simulink model "BMS_Advanced_Protection_Algorithm_Design"  (R2024a)
settings: Solver=VariableStepAuto  StartTime=0.0  StopTime=inf  RelTol=1e-3
libraries: simulink x3
settings Model: Creator=gopin  LastModifiedBy=gopin

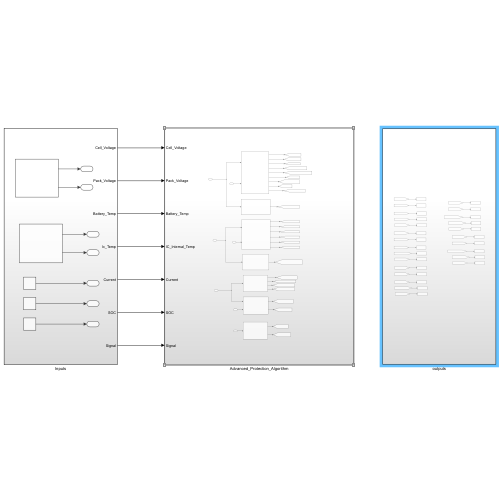
[thumbnail: Simulink's stored preview of the top-level diagram]
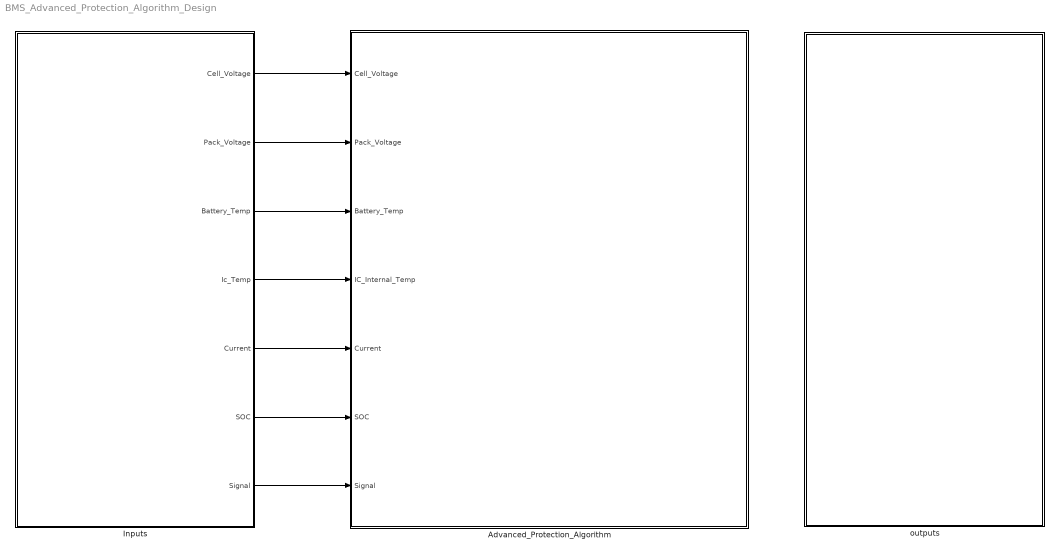
== system BMS_Advanced_Protection_Algorithm_Design ==
  Advanced_Protection_Algorithm : Subsystem
  Inputs : Subsystem
  outputs : Subsystem
  wires:
  Inputs/1(Cell_Voltage) -> Advanced_Protection_Algorithm/1(Cell_Voltage)
  Inputs/2(Pack_Voltage) -> Advanced_Protection_Algorithm/2(Pack_Voltage)
  Inputs/3(Battery_Temp) -> Advanced_Protection_Algorithm/3(Battery_Temp)
  Inputs/4(Ic_Temp) -> Advanced_Protection_Algorithm/4(IC_Internal_Temp)
  Inputs/5(Current) -> Advanced_Protection_Algorithm/5(Current)
  Inputs/6(SOC) -> Advanced_Protection_Algorithm/6(SOC)
  Inputs/7(Signal) -> Advanced_Protection_Algorithm/7(Signal)

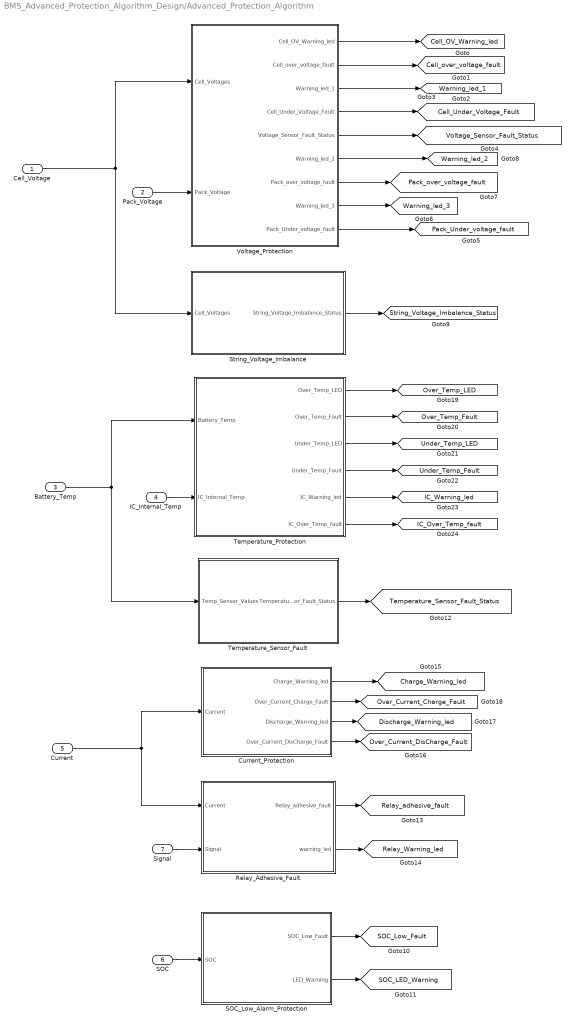
== system BMS_Advanced_Protection_Algorithm_Design/Advanced_Protection_Algorithm ==
  Cell_Voltage : Inport
  Pack_Voltage : Inport  Port=2
  Battery_Temp : Inport  Port=3
  IC_Internal_Temp : Inport  Port=4
  Current : Inport  Port=5
  SOC : Inport  Port=6
  Signal : Inport  Port=7
  Current_Protection : Subsystem
  Relay_Adhesive_Fault : Subsystem
  SOC_Low_Alarm_Protection : Subsystem
  String_Voltage_Imbalance : Subsystem
  Temperature_Protection : Subsystem
  Temperature_Sensor_Fault : Subsystem
  Voltage_Protection : Subsystem
  tag scope: Cell_OV_Warning_led=global, Cell_Under_Voltage_Fault=global, Cell_over_voltage_fault=global, Charge_Warning_led=global, Discharge_Warning_led=global, IC_Over_Temp_fault=global, IC_Warning_led=global, Over_Current_Charge_Fault=global, Over_Current_DisCharge_Fault=global, Over_Temp_Fault=global, Over_Temp_LED=global, Pack_Under_voltage_fault=global, Pack_over_voltage_fault=global, Relay_Warning_led=global, Relay_adhesive_fault=global, SOC_LED_Warning=global, SOC_Low_Fault=global, String_Voltage_Imbalance_Status=global, Temperature_Sensor_Fault_Status=global, Under_Temp_Fault=global, Under_Temp_LED=global, Voltage_Sensor_Fault_Status=global, Warning_led_1=global, Warning_led_2=global, Warning_led_3=global
  wires:
  Current_Protection/4(Over_Current_DisCharge_Fault) -> [Over_Current_DisCharge_Fault]
  Temperature_Protection/4(Under_Temp_Fault) -> [Under_Temp_Fault]
  Signal/1 -> Relay_Adhesive_Fault/2(Signal)
  Current/1 -> Current_Protection/1(Current), Relay_Adhesive_Fault/1(Current)
  Temperature_Sensor_Fault/1(Temperature_Sensor_Fault_Status) -> [Temperature_Sensor_Fault_Status]
  Relay_Adhesive_Fault/1(Relay_adhesive_fault) -> [Relay_adhesive_fault]
  Temperature_Protection/1(Over_Temp_LED) -> [Over_Temp_LED]
  Relay_Adhesive_Fault/2(warning_led) -> [Relay_Warning_led]
  Current_Protection/2(Over_Current_Charge_Fault) -> [Over_Current_Charge_Fault]
  Cell_Voltage/1 -> Voltage_Protection/1(Cell_Voltages), String_Voltage_Imbalance/1(Cell_Voltages)
  Pack_Voltage/1 -> Voltage_Protection/2(Pack_Voltage)
  Temperature_Protection/2(Over_Temp_Fault) -> [Over_Temp_Fault]
  String_Voltage_Imbalance/1(String_Voltage_Imbalance_Status) -> [String_Voltage_Imbalance_Status]
  SOC_Low_Alarm_Protection/1(SOC_Low_Fault) -> [SOC_Low_Fault]
  SOC/1 -> SOC_Low_Alarm_Protection/1(SOC)
  IC_Internal_Temp/1 -> Temperature_Protection/2(IC_Internal_Temp)
  Temperature_Protection/3(Under_Temp_LED) -> [Under_Temp_LED]
  SOC_Low_Alarm_Protection/2(LED_Warning) -> [SOC_LED_Warning]
  Current_Protection/3(Discharge_Warning_led) -> [Discharge_Warning_led]
  Voltage_Protection/1(Cell_OV_Warning_led) -> [Cell_OV_Warning_led]
  Voltage_Protection/3(Warning_led_1) -> [Warning_led_1]
  Voltage_Protection/5(Voltage_Sensor_Fault_Status) -> [Voltage_Sensor_Fault_Status]
  Voltage_Protection/6(Warning_led_2) -> [Warning_led_2]
  Voltage_Protection/7(Pack_over_voltage_fault) -> [Pack_over_voltage_fault]
  Voltage_Protection/8(Warning_led_3) -> [Warning_led_3]
  Temperature_Protection/5(IC_Warning_led) -> [IC_Warning_led]
  Temperature_Protection/6(IC_Over_Temp_fault) -> [IC_Over_Temp_fault]
  Battery_Temp/1 -> Temperature_Protection/1(Battery_Temp), Temperature_Sensor_Fault/1(Temp_Sensor_Values)
  Voltage_Protection/2(Cell_over_voltage_fault) -> [Cell_over_voltage_fault]
  Voltage_Protection/4(Cell_Under_Voltage_Fault) -> [Cell_Under_Voltage_Fault]
  Voltage_Protection/9(Pack_Under_voltage_fault) -> [Pack_Under_voltage_fault]
  Current_Protection/1(Charge_Warning_led) -> [Charge_Warning_led]

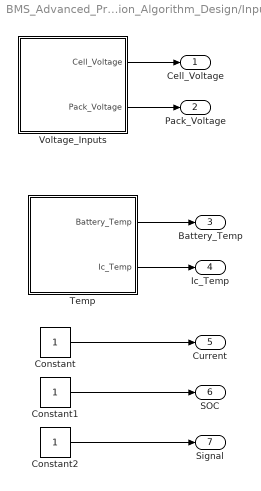
== system BMS_Advanced_Protection_Algorithm_Design/Inputs ==
  Constant : Constant
  Constant1 : Constant
  Constant2 : Constant
  Temp : Subsystem
  Voltage_Inputs : Subsystem
  Cell_Voltage : Outport
  Pack_Voltage : Outport  Port=2
  Battery_Temp : Outport  Port=3
  Ic_Temp : Outport  Port=4
  Current : Outport  Port=5
  SOC : Outport  Port=6
  Signal : Outport  Port=7
  wires:
  Voltage_Inputs/1(Cell_Voltage) -> Cell_Voltage/1
  Voltage_Inputs/2(Pack_Voltage) -> Pack_Voltage/1
  Temp/1(Battery_Temp) -> Battery_Temp/1
  Temp/2(Ic_Temp) -> Ic_Temp/1
  Constant/1 -> Current/1
  Constant1/1 -> SOC/1
  Constant2/1 -> Signal/1

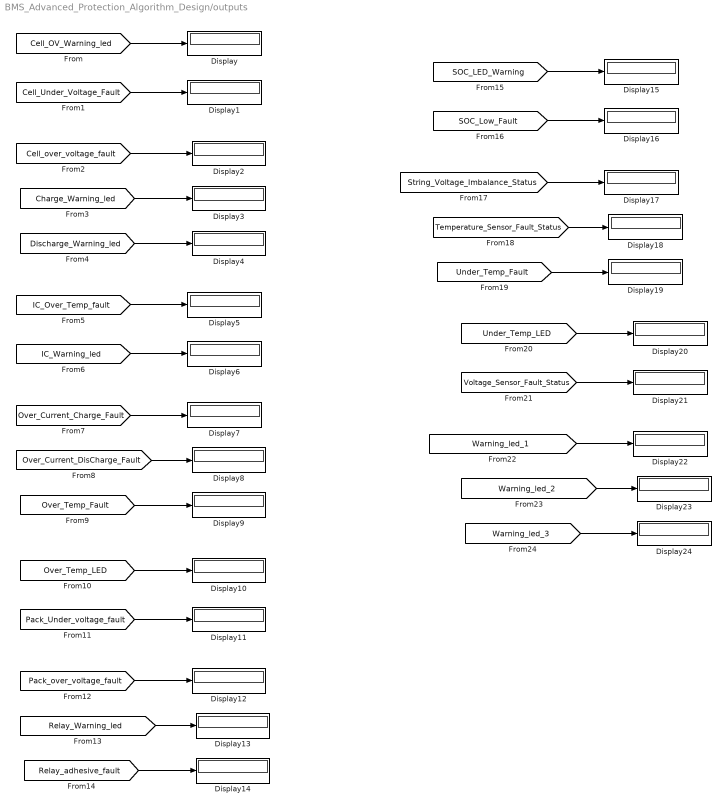
== system BMS_Advanced_Protection_Algorithm_Design/outputs ==
  Display{,1..24} (25 alike) : Display
  wires:
  [Cell_OV_Warning_led] -> Display/1
  [Cell_Under_Voltage_Fault] -> Display1/1
  [Cell_over_voltage_fault] -> Display2/1
  [Charge_Warning_led] -> Display3/1
  [Discharge_Warning_led] -> Display4/1
  [IC_Warning_led] -> Display6/1
  [Over_Current_Charge_Fault] -> Display7/1
  [Over_Current_DisCharge_Fault] -> Display8/1
  [Over_Temp_Fault] -> Display9/1
  [IC_Over_Temp_fault] -> Display5/1
  [Relay_adhesive_fault] -> Display14/1
  [Relay_Warning_led] -> Display13/1
  [Pack_over_voltage_fault] -> Display12/1
  [Over_Temp_LED] -> Display10/1
  [Pack_Under_voltage_fault] -> Display11/1
  [SOC_LED_Warning] -> Display15/1
  [String_Voltage_Imbalance_Status] -> Display17/1
  [Under_Temp_Fault] -> Display19/1
  [SOC_Low_Fault] -> Display16/1
  [Temperature_Sensor_Fault_Status] -> Display18/1
  [Warning_led_2] -> Display23/1
  [Warning_led_1] -> Display22/1
  [Voltage_Sensor_Fault_Status] -> Display21/1
  [Warning_led_3] -> Display24/1
  [Under_Temp_LED] -> Display20/1

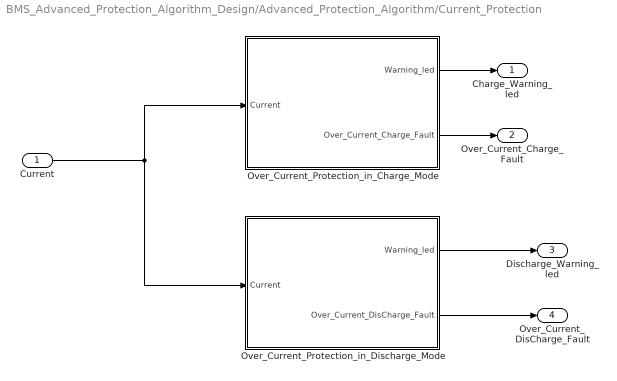
== system BMS_Advanced_Protection_Algorithm_Design/Advanced_Protection_Algorithm/Current_Protection ==
  Current : Inport
  Over_Current_Protection_in_Charge_Mode : Subsystem
  Over_Current_Protection_in_Discharge_Mode : Subsystem
  Charge_Warning_led : Outport
  Over_Current_Charge_Fault : Outport  Port=2
  Discharge_Warning_led : Outport  Port=3
  Over_Current_DisCharge_Fault : Outport  Port=4
  wires:
  Over_Current_Protection_in_Charge_Mode/1(Warning_led) -> Charge_Warning_led/1
  Over_Current_Protection_in_Charge_Mode/2(Over_Current_Charge_Fault) -> Over_Current_Charge_Fault/1
  Over_Current_Protection_in_Discharge_Mode/2(Over_Current_DisCharge_Fault) -> Over_Current_DisCharge_Fault/1
  Over_Current_Protection_in_Discharge_Mode/1(Warning_led) -> Discharge_Warning_led/1
  Current/1 -> Over_Current_Protection_in_Discharge_Mode/1(Current), Over_Current_Protection_in_Charge_Mode/1(Current)

== system BMS_Advanced_Protection_Algorithm_Design/Advanced_Protection_Algorithm/Relay_Adhesive_Fault ==
  Current : Inport
  Signal : Inport  Port=2
  Chart : Stateflow chart  TreatAsAtomicUnit=on
  Relay_adhesive_fault : Outport
  warning_led : Outport  Port=2
  wires:
  Current/1 -> Chart/1(Current)
  Signal/1 -> Chart/2(Signal)
  Chart/1(relay_adhesive_fault) -> Relay_adhesive_fault/1
  Chart/2(warning_led) -> warning_led/1

== system BMS_Advanced_Protection_Algorithm_Design/Advanced_Protection_Algorithm/SOC_Low_Alarm_Protection ==
  SOC : Inport
  Chart : Stateflow chart  TreatAsAtomicUnit=on
  SOC_Low_Fault : Outport
  LED_Warning : Outport  Port=2
  wires:
  Chart/1(SOC_Low_Fault) -> SOC_Low_Fault/1
  SOC/1 -> Chart/1(SOC)
  Chart/2(warning_led) -> LED_Warning/1

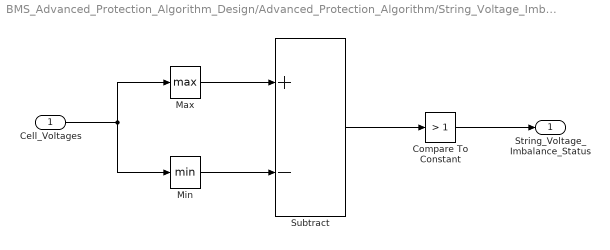
== system BMS_Advanced_Protection_Algorithm_Design/Advanced_Protection_Algorithm/String_Voltage_Imbalance ==
  Cell_Voltages : Inport
  Compare To Constant : simulink/Logic and Bit Operations/Compare To Constant  relop=>  const=1  OutDataTypeStr=boolean
  Max : MinMax  Function=max
  Min : MinMax
  Subtract : Sum  Inputs=+-
  String_Voltage_Imbalance_Status : Outport
  wires:
  Subtract/1 -> Compare To Constant/1
  Compare To Constant/1 -> String_Voltage_Imbalance_Status/1
  Min/1 -> Subtract/2
  Max/1 -> Subtract/1
  Cell_Voltages/1 -> Min/1, Max/1

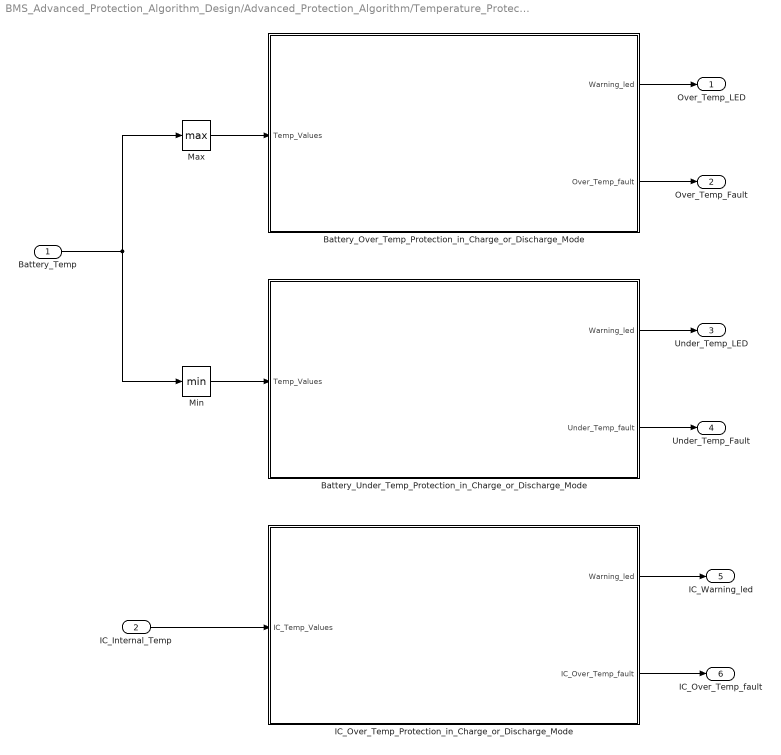
== system BMS_Advanced_Protection_Algorithm_Design/Advanced_Protection_Algorithm/Temperature_Protection ==
  Battery_Temp : Inport
  IC_Internal_Temp : Inport  Port=2
  Battery_Over_Temp_Protection_in_Charge_or_Discharge_Mode : Subsystem
  Battery_Under_Temp_Protection_in_Charge_or_Discharge_Mode : Subsystem
  IC_Over_Temp_Protection_in_Charge_or_Discharge_Mode : Subsystem
  Max : MinMax  Function=max
  Min : MinMax
  Over_Temp_LED : Outport
  Over_Temp_Fault : Outport  Port=2
  Under_Temp_LED : Outport  Port=3
  Under_Temp_Fault : Outport  Port=4
  IC_Warning_led : Outport  Port=5
  IC_Over_Temp_fault : Outport  Port=6
  wires:
  Battery_Over_Temp_Protection_in_Charge_or_Discharge_Mode/1(Warning_led) -> Over_Temp_LED/1
  Battery_Over_Temp_Protection_in_Charge_or_Discharge_Mode/2(Over_Temp_fault) -> Over_Temp_Fault/1
  Max/1 -> Battery_Over_Temp_Protection_in_Charge_or_Discharge_Mode/1(Temp_Values)
  Min/1 -> Battery_Under_Temp_Protection_in_Charge_or_Discharge_Mode/1(Temp_Values)
  Battery_Temp/1 -> Min/1, Max/1
  Battery_Under_Temp_Protection_in_Charge_or_Discharge_Mode/1(Warning_led) -> Under_Temp_LED/1
  Battery_Under_Temp_Protection_in_Charge_or_Discharge_Mode/2(Under_Temp_fault) -> Under_Temp_Fault/1
  IC_Internal_Temp/1 -> IC_Over_Temp_Protection_in_Charge_or_Discharge_Mode/1(IC_Temp_Values)
  IC_Over_Temp_Protection_in_Charge_or_Discharge_Mode/1(Warning_led) -> IC_Warning_led/1
  IC_Over_Temp_Protection_in_Charge_or_Discharge_Mode/2(IC_Over_Temp_fault) -> IC_Over_Temp_fault/1

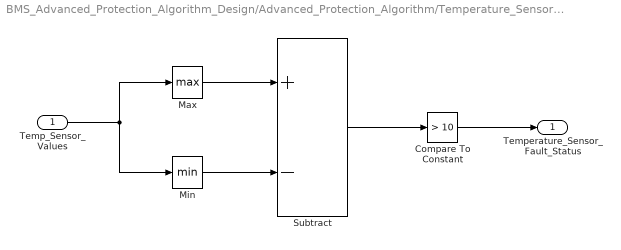
== system BMS_Advanced_Protection_Algorithm_Design/Advanced_Protection_Algorithm/Temperature_Sensor_Fault ==
  Temp_Sensor_Values : Inport
  Compare To Constant : simulink/Logic and Bit Operations/Compare To Constant  relop=>  const=10  OutDataTypeStr=boolean
  Max : MinMax  Function=max
  Min : MinMax
  Subtract : Sum  Inputs=+-
  Temperature_Sensor_Fault_Status : Outport
  wires:
  Temp_Sensor_Values/1 -> Min/1, Max/1
  Max/1 -> Subtract/1
  Min/1 -> Subtract/2
  Subtract/1 -> Compare To Constant/1
  Compare To Constant/1 -> Temperature_Sensor_Fault_Status/1

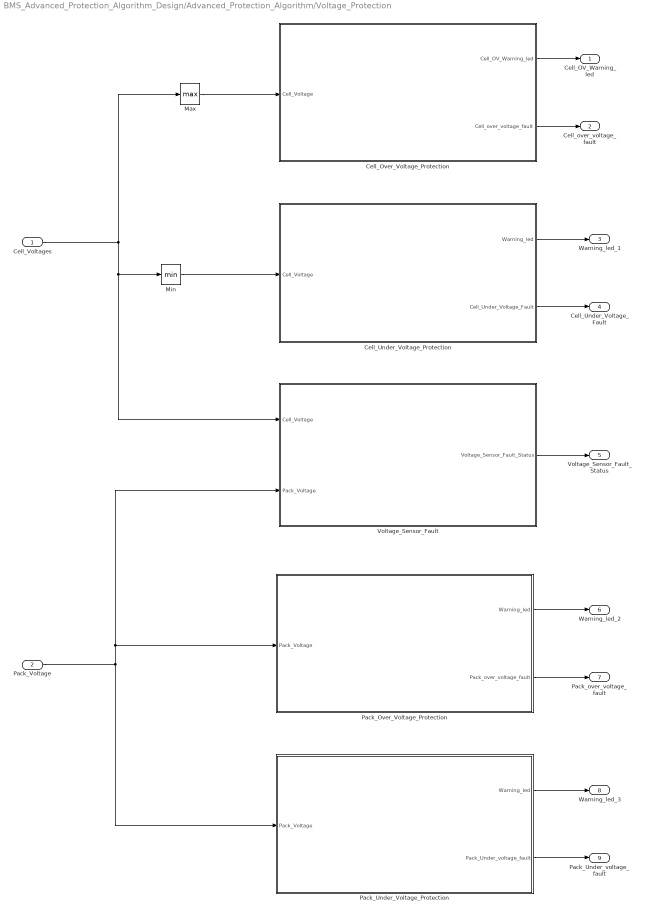
== system BMS_Advanced_Protection_Algorithm_Design/Advanced_Protection_Algorithm/Voltage_Protection ==
  Cell_Voltages : Inport
  Pack_Voltage : Inport  Port=2
  Cell_Over_Voltage_Protection : Subsystem
  Cell_Under_Voltage_Protection : Subsystem
  Max : MinMax  Function=max
  Min : MinMax
  Pack_Over_Voltage_Protection : Subsystem
  Pack_Under_Voltage_Protection : Subsystem
  Voltage_Sensor_Fault : Subsystem
  Cell_OV_Warning_led : Outport
  Cell_over_voltage_fault : Outport  Port=2
  Warning_led_1 : Outport  Port=3
  Cell_Under_Voltage_Fault : Outport  Port=4
  Voltage_Sensor_Fault_Status : Outport  Port=5
  Warning_led_2 : Outport  Port=6
  Pack_over_voltage_fault : Outport  Port=7
  Warning_led_3 : Outport  Port=8
  Pack_Under_voltage_fault : Outport  Port=9
  wires:
  Max/1 -> Cell_Over_Voltage_Protection/1(Cell_Voltage)
  Min/1 -> Cell_Under_Voltage_Protection/1(Cell_Voltage)
  Cell_Voltages/1 -> Max/1, Voltage_Sensor_Fault/1(Cell_Voltage), Min/1
  Pack_Voltage/1 -> Pack_Under_Voltage_Protection/1(Pack_Voltage), Pack_Over_Voltage_Protection/1(Pack_Voltage), Voltage_Sensor_Fault/2(Pack_Voltage)
  Cell_Over_Voltage_Protection/1(Cell_OV_Warning_led) -> Cell_OV_Warning_led/1
  Cell_Over_Voltage_Protection/2(Cell_over_voltage_fault) -> Cell_over_voltage_fault/1
  Cell_Under_Voltage_Protection/1(Warning_led) -> Warning_led_1/1
  Cell_Under_Voltage_Protection/2(Cell_Under_Voltage_Fault) -> Cell_Under_Voltage_Fault/1
  Voltage_Sensor_Fault/1(Voltage_Sensor_Fault_Status) -> Voltage_Sensor_Fault_Status/1
  Pack_Over_Voltage_Protection/1(Warning_led) -> Warning_led_2/1
  Pack_Over_Voltage_Protection/2(Pack_over_voltage_fault) -> Pack_over_voltage_fault/1
  Pack_Under_Voltage_Protection/1(Warning_led) -> Warning_led_3/1
  Pack_Under_Voltage_Protection/2(Pack_Under_voltage_fault) -> Pack_Under_voltage_fault/1

== system BMS_Advanced_Protection_Algorithm_Design/Inputs/Temp ==
  Battery_Temperature : Subsystem
  Constant : Constant
  Mux : Mux  Inputs=7
  Battery_Temp : Outport
  Ic_Temp : Outport  Port=2
  wires:
  Mux/1 -> Battery_Temp/1
  Battery_Temperature/1(Outport) -> Mux/1
  Battery_Temperature/2(Outport1) -> Mux/2
  Battery_Temperature/3(Outport2) -> Mux/3
  Battery_Temperature/4(Outport3) -> Mux/4
  Battery_Temperature/5(Outport4) -> Mux/5
  Battery_Temperature/6(Outport5) -> Mux/6
  Battery_Temperature/7(Outport6) -> Mux/7
  Constant/1 -> Ic_Temp/1

== system BMS_Advanced_Protection_Algorithm_Design/Inputs/Voltage_Inputs ==
  Cell_Voltages : Subsystem
  Constant : Constant
  Mux : Mux  Inputs=14
  Cell_Voltage : Outport
  Pack_Voltage : Outport  Port=2
  wires:
  Constant/1 -> Pack_Voltage/1
  Mux/1 -> Cell_Voltage/1
  Cell_Voltages/1(Outport) -> Mux/1
  Cell_Voltages/2(Outport1) -> Mux/2
  Cell_Voltages/3(Outport2) -> Mux/3
  Cell_Voltages/4(Outport3) -> Mux/4
  Cell_Voltages/5(Outport4) -> Mux/5
  Cell_Voltages/6(Outport5) -> Mux/6
  Cell_Voltages/7(Outport6) -> Mux/7
  Cell_Voltages/8(Outport7) -> Mux/8
  Cell_Voltages/9(Outport8) -> Mux/9
  Cell_Voltages/10(Outport9) -> Mux/10
  Cell_Voltages/11(Outport10) -> Mux/11
  Cell_Voltages/12(Outport11) -> Mux/12
  Cell_Voltages/13(Outport12) -> Mux/13
  Cell_Voltages/14(Outport13) -> Mux/14

== system BMS_Advanced_Protection_Algorithm_Design/Advanced_Protection_Algorithm/Current_Protection/Over_Current_Protection_in_Charge_Mode ==
  Current : Inport
  Over_Current_Protection_in_Charge_Mode : Stateflow chart  TreatAsAtomicUnit=on
  Warning_led : Outport
  Over_Current_Charge_Fault : Outport  Port=2
  wires:
  Current/1 -> Over_Current_Protection_in_Charge_Mode/1(Current)
  Over_Current_Protection_in_Charge_Mode/1(Warning_led) -> Warning_led/1
  Over_Current_Protection_in_Charge_Mode/2(Over_Current_Charge_Fault) -> Over_Current_Charge_Fault/1

== system BMS_Advanced_Protection_Algorithm_Design/Advanced_Protection_Algorithm/Current_Protection/Over_Current_Protection_in_Discharge_Mode ==
  Current : Inport
  Over_Current_Protection_in_DisCharge_Mode : Stateflow chart  TreatAsAtomicUnit=on
  Warning_led : Outport
  Over_Current_DisCharge_Fault : Outport  Port=2
  wires:
  Current/1 -> Over_Current_Protection_in_DisCharge_Mode/1(Current)
  Over_Current_Protection_in_DisCharge_Mode/1(Warning_led) -> Warning_led/1
  Over_Current_Protection_in_DisCharge_Mode/2(Over_Current_DisCharge_Fault) -> Over_Current_DisCharge_Fault/1

== system BMS_Advanced_Protection_Algorithm_Design/Advanced_Protection_Algorithm/Temperature_Protection/Battery_Over_Temp_Protection_in_Charge_or_Discharge_Mode ==
  Temp_Values : Inport
  Over_Temp_Protection : Stateflow chart  TreatAsAtomicUnit=on
  Warning_led : Outport
  Over_Temp_fault : Outport  Port=2
  wires:
  Over_Temp_Protection/1(Warning_led) -> Warning_led/1
  Temp_Values/1 -> Over_Temp_Protection/1(Max_Temp_data)
  Over_Temp_Protection/2(Over_Temp_fault) -> Over_Temp_fault/1

== system BMS_Advanced_Protection_Algorithm_Design/Advanced_Protection_Algorithm/Temperature_Protection/Battery_Under_Temp_Protection_in_Charge_or_Discharge_Mode ==
  Temp_Values : Inport
  Under_Temp_Protection : Stateflow chart  TreatAsAtomicUnit=on
  Warning_led : Outport
  Under_Temp_fault : Outport  Port=2
  wires:
  Under_Temp_Protection/1(Warning_led) -> Warning_led/1
  Temp_Values/1 -> Under_Temp_Protection/1(Min_Temp_data)
  Under_Temp_Protection/2(Under_Temp_fault) -> Under_Temp_fault/1

== system BMS_Advanced_Protection_Algorithm_Design/Advanced_Protection_Algorithm/Temperature_Protection/IC_Over_Temp_Protection_in_Charge_or_Discharge_Mode ==
  IC_Temp_Values : Inport
  IC_Over_Temp_Protection : Stateflow chart  TreatAsAtomicUnit=on
  Warning_led : Outport
  IC_Over_Temp_fault : Outport  Port=2
  wires:
  IC_Over_Temp_Protection/1(Warning_led) -> Warning_led/1
  IC_Over_Temp_Protection/2(IC_Over_Temp_fault) -> IC_Over_Temp_fault/1
  IC_Temp_Values/1 -> IC_Over_Temp_Protection/1(IC_Temp_data)

== system BMS_Advanced_Protection_Algorithm_Design/Advanced_Protection_Algorithm/Voltage_Protection/Cell_Over_Voltage_Protection ==
  Cell_Voltage : Inport
  Over_Voltage_Protection : Stateflow chart  TreatAsAtomicUnit=on
  Cell_OV_Warning_led : Outport
  Cell_over_voltage_fault : Outport  Port=2
  wires:
  Cell_Voltage/1 -> Over_Voltage_Protection/1(Cell_Voltage)
  Over_Voltage_Protection/2(Cell_over_voltage_fault) -> Cell_over_voltage_fault/1
  Over_Voltage_Protection/1(Warning_led) -> Cell_OV_Warning_led/1

== system BMS_Advanced_Protection_Algorithm_Design/Advanced_Protection_Algorithm/Voltage_Protection/Cell_Under_Voltage_Protection ==
  Cell_Voltage : Inport
  Under_Voltage_Protection : Stateflow chart  TreatAsAtomicUnit=on
  Warning_led : Outport
  Cell_Under_Voltage_Fault : Outport  Port=2
  wires:
  Cell_Voltage/1 -> Under_Voltage_Protection/1(Cell_Voltage)
  Under_Voltage_Protection/1(Warning_led) -> Warning_led/1
  Under_Voltage_Protection/2(Cell_Under_voltage_fault) -> Cell_Under_Voltage_Fault/1

== system BMS_Advanced_Protection_Algorithm_Design/Advanced_Protection_Algorithm/Voltage_Protection/Pack_Over_Voltage_Protection ==
  Pack_Voltage : Inport
  Over_Voltage_Protection : Stateflow chart  TreatAsAtomicUnit=on
  Warning_led : Outport
  Pack_over_voltage_fault : Outport  Port=2
  wires:
  Over_Voltage_Protection/1(Warning_led) -> Warning_led/1
  Pack_Voltage/1 -> Over_Voltage_Protection/1(Pack_Voltage)
  Over_Voltage_Protection/2(Pack_over_voltage_fault) -> Pack_over_voltage_fault/1

== system BMS_Advanced_Protection_Algorithm_Design/Advanced_Protection_Algorithm/Voltage_Protection/Pack_Under_Voltage_Protection ==
  Pack_Voltage : Inport
  Under_Voltage_Protection : Stateflow chart  TreatAsAtomicUnit=on
  Warning_led : Outport
  Pack_Under_voltage_fault : Outport  Port=2
  wires:
  Under_Voltage_Protection/1(Warning_led) -> Warning_led/1
  Pack_Voltage/1 -> Under_Voltage_Protection/1(Pack_Voltage)
  Under_Voltage_Protection/2(Pack_Under_voltage_fault) -> Pack_Under_voltage_fault/1

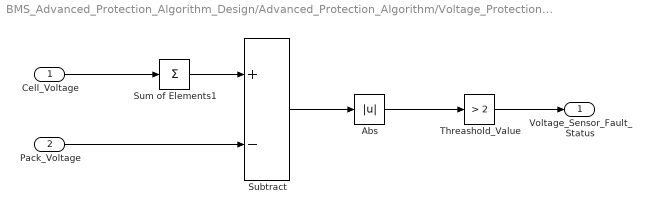
== system BMS_Advanced_Protection_Algorithm_Design/Advanced_Protection_Algorithm/Voltage_Protection/Voltage_Sensor_Fault ==
  Cell_Voltage : Inport
  Pack_Voltage : Inport  Port=2
  Abs : Abs  SaturateOnIntegerOverflow=off
  Subtract : Sum  Inputs=+-
  Sum of Elements1 : Sum  Inputs=+
  Threashold_Value : simulink/Logic and Bit Operations/Compare To Constant  relop=>  const=2  OutDataTypeStr=boolean
  Voltage_Sensor_Fault_Status : Outport
  wires:
  Cell_Voltage/1 -> Sum of Elements1/1
  Pack_Voltage/1 -> Subtract/2
  Sum of Elements1/1 -> Subtract/1
  Subtract/1 -> Abs/1
  Abs/1 -> Threashold_Value/1
  Threashold_Value/1 -> Voltage_Sensor_Fault_Status/1

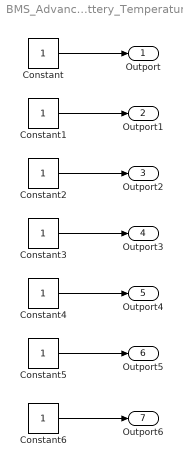
== system BMS_Advanced_Protection_Algorithm_Design/Inputs/Temp/Battery_Temperature ==
  Constant{,1..6} (7 alike) : Constant
  Outport : Outport
  Outport1 : Outport  Port=2
  Outport2 : Outport  Port=3
  Outport3 : Outport  Port=4
  Outport4 : Outport  Port=5
  Outport5 : Outport  Port=6
  Outport6 : Outport  Port=7
  wires:
  Constant/1 -> Outport/1
  Constant1/1 -> Outport1/1
  Constant2/1 -> Outport2/1
  Constant3/1 -> Outport3/1
  Constant4/1 -> Outport4/1
  Constant5/1 -> Outport5/1
  Constant6/1 -> Outport6/1

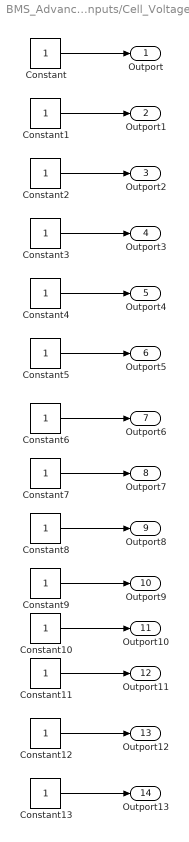
== system BMS_Advanced_Protection_Algorithm_Design/Inputs/Voltage_Inputs/Cell_Voltages ==
  Constant{,1..13} (14 alike) : Constant
  Outport : Outport
  Outport1 : Outport  Port=2
  Outport2 : Outport  Port=3
  Outport3 : Outport  Port=4
  Outport4 : Outport  Port=5
  Outport5 : Outport  Port=6
  Outport6 : Outport  Port=7
  Outport7 : Outport  Port=8
  Outport8 : Outport  Port=9
  Outport9 : Outport  Port=10
  Outport10 : Outport  Port=11
  Outport11 : Outport  Port=12
  Outport12 : Outport  Port=13
  Outport13 : Outport  Port=14
  wires:
  Constant/1 -> Outport/1
  Constant1/1 -> Outport1/1
  Constant2/1 -> Outport2/1
  Constant3/1 -> Outport3/1
  Constant4/1 -> Outport4/1
  Constant5/1 -> Outport5/1
  Constant6/1 -> Outport6/1
  Constant7/1 -> Outport7/1
  Constant8/1 -> Outport8/1
  Constant9/1 -> Outport9/1
  Constant10/1 -> Outport10/1
  Constant11/1 -> Outport11/1
  Constant12/1 -> Outport12/1
  Constant13/1 -> Outport13/1

== stateflow chart BMS_Advanced_Protection_Algorithm_Design/Advanced_Protection_Algorithm/Temperature_Protection/Battery_Over_Temp_Protection_in_Charge_or_Discharge_Mode/Over_Temp_Protection ==
  state Initial_Condition
    en:
    Over_Temp_fault=0;
    Warning_led=0;
  state Level_1_Trigger
    en:
    Over_Temp_fault=1;
    state LED_off
      en:
      Warning_led=0;
    state LED_on
      en:
      Warning_led=1;
    (default) -> LED_off
    LED_off -> LED_on : [after(1,sec)]
    LED_on -> LED_off : [after(1,sec)]
  state Level_3_Trigger
    en:
    Over_Temp_fault=1;
    Warning_led=1;
    du:
    Warning_led=1;
  (default) -> Initial_Condition
  Initial_Condition -> Level_1_Trigger : [Max_Temp_data > 55 && after(5,sec)]
  Level_1_Trigger -> Initial_Condition [order 1] : [Max_Temp_data < 50]
  Level_3_Trigger -> Initial_Condition [order 2] : [Max_Temp_data<50]
  Level_1_Trigger -> Level_3_Trigger [order 2] : [Max_Temp_data>60 && after(3,sec)]
  Level_3_Trigger -> Level_1_Trigger [order 1] : [Max_Temp_data<60]
  data: Warning_led output; Max_Temp_data input; Over_Temp_fault output

== stateflow chart BMS_Advanced_Protection_Algorithm_Design/Advanced_Protection_Algorithm/Temperature_Protection/Battery_Under_Temp_Protection_in_Charge_or_Discharge_Mode/Under_Temp_Protection ==
  state Initial_Condition
    en:
    Under_Temp_fault=0;
    Warning_led=0;
  state Level_1_Trigger
    en:
    Under_Temp_fault=1;
    state LED_off
      en:
      Warning_led=0;
    state LED_on
      en:
      Warning_led=1;
    (default) -> LED_off
    LED_off -> LED_on : [after(1,sec)]
    LED_on -> LED_off : [after(1,sec)]
  state Level_3_Trigger
    en:
    Under_Temp_fault=1;
    Warning_led=1;
    du:
    Warning_led=1;
  (default) -> Initial_Condition
  Initial_Condition -> Level_1_Trigger : [Min_Temp_data < 15 && after(5,sec)]
  Level_1_Trigger -> Initial_Condition [order 1] : [Min_Temp_data > 20]
  Level_3_Trigger -> Initial_Condition [order 2] : [Min_Temp_data>20]
  Level_1_Trigger -> Level_3_Trigger [order 2] : [Min_Temp_data <10 && after(3,sec)]
  Level_3_Trigger -> Level_1_Trigger [order 1] : [Min_Temp_data> 10]
  data: Warning_led output; Min_Temp_data input; Under_Temp_fault output

== stateflow chart BMS_Advanced_Protection_Algorithm_Design/Advanced_Protection_Algorithm/Temperature_Protection/IC_Over_Temp_Protection_in_Charge_or_Discharge_Mode/IC_Over_Temp_Protection ==
  state Initial_Condition
    en:
    IC_Over_Temp_fault=0;
    Warning_led=0;
  state Level_1_Trigger
    en:
    IC_Over_Temp_fault=1;
    state LED_off
      en:
      Warning_led=0;
    state LED_on
      en:
      Warning_led=1;
    (default) -> LED_off
    LED_off -> LED_on : [after(1,sec)]
    LED_on -> LED_off : [after(1,sec)]
  state Level_3_Trigger
    en:
    IC_Over_Temp_fault=1;
    Warning_led=1;
    du:
    Warning_led=1;
  (default) -> Initial_Condition
  Initial_Condition -> Level_1_Trigger : [IC_Temp_data > 60 && after(5,sec)]
  Level_1_Trigger -> Initial_Condition [order 1] : [IC_Temp_data < 55]
  Level_3_Trigger -> Initial_Condition [order 2] : [IC_Temp_data<55]
  Level_1_Trigger -> Level_3_Trigger [order 2] : [IC_Temp_data>70 && after(3,sec)]
  Level_3_Trigger -> Level_1_Trigger [order 1] : [IC_Temp_data<70]
  data: Warning_led output; IC_Over_Temp_fault output; IC_Temp_data input

== stateflow chart BMS_Advanced_Protection_Algorithm_Design/Advanced_Protection_Algorithm/SOC_Low_Alarm_Protection/Chart ==
  state Initial_Condition
    en:
    SOC_Low_Fault=0;
  state Level_1_Warning
    en:
    SOC_Low_Fault=1;
    state LED_off
      en:
      warning_led=0;
    state LED_on
      en:
      warning_led=1;
    (default) -> LED_off
    LED_on -> LED_off : [after(1,sec)]
    LED_off -> LED_on : [after(1,sec)]
  (default) -> Initial_Condition
  Initial_Condition -> Level_1_Warning : [SOC < 10 && after(5,sec)]
  Level_1_Warning -> Initial_Condition : [SOC >10]
  data: SOC_Low_Fault output; warning_led output; SOC input

== stateflow chart BMS_Advanced_Protection_Algorithm_Design/Advanced_Protection_Algorithm/Current_Protection/Over_Current_Protection_in_Charge_Mode/Over_Current_Protection_in_Charge_Mode ==
  state Initial_Condition
    en:
    Over_Current_Charge_Fault=0;
    Warning_led=0;
  state Level_1_Trigger
    en:
    Over_Current_Charge_Fault=1;
    state LED_off
      en:
      Warning_led=0;
    state LED_on
      en:
      Warning_led=1;
    (default) -> LED_off
    LED_off -> LED_on : [after(1,sec)]
    LED_on -> LED_off : [after(1,sec)]
  state Level_3_Trigger
    en:
    Over_Current_Charge_Fault=1;
    Warning_led=1;
    du:
    Warning_led=1;
  (default) -> Initial_Condition
  Initial_Condition -> Level_1_Trigger : [Current > 3 && after(5,sec)]
  Level_1_Trigger -> Initial_Condition [order 1] : [Current < 3]
  Level_3_Trigger -> Initial_Condition [order 2] : [Current < 3]
  Level_1_Trigger -> Level_3_Trigger [order 2] : [Current >4 && after(3,sec)]
  Level_3_Trigger -> Level_1_Trigger [order 1] : [Current <4]
  data: Warning_led output; Over_Current_Charge_Fault output; Current input

== stateflow chart BMS_Advanced_Protection_Algorithm_Design/Advanced_Protection_Algorithm/Current_Protection/Over_Current_Protection_in_Discharge_Mode/Over_Current_Protection_in_DisCharge_Mode ==
  state Initial_Condition
    en:
    Over_Current_DisCharge_Fault=0;
    Warning_led=0;
  state Level_1_Trigger
    en:
    Over_Current_DisCharge_Fault=1;
    state LED_off
      en:
      Warning_led=0;
    state LED_on
      en:
      Warning_led=1;
    (default) -> LED_off
    LED_off -> LED_on : [after(1,sec)]
    LED_on -> LED_off : [after(1,sec)]
  state Level_3_Trigger
    en:
    Over_Current_DisCharge_Fault=1;
    Warning_led=1;
    du:
    Warning_led=1;
  (default) -> Initial_Condition
  Initial_Condition -> Level_1_Trigger : [Current < -5 && after(5,sec)]
  Level_1_Trigger -> Initial_Condition [order 1] : [Current >-5]
  Level_3_Trigger -> Initial_Condition [order 2] : [Current >-5]
  Level_1_Trigger -> Level_3_Trigger [order 2] : [Current < -6 && after(3,sec)]
  Level_3_Trigger -> Level_1_Trigger [order 1] : [Current > -6]
  data: Warning_led output; Current input; Over_Current_DisCharge_Fault output

== stateflow chart BMS_Advanced_Protection_Algorithm_Design/Advanced_Protection_Algorithm/Relay_Adhesive_Fault/Chart ==
  state Cond_1
    en:
    relay_adhesive_fault=0;
  state Cond_2
    en:
    relay_adhesive_fault=1;
    state Led_off
      en:
      warning_led=0;
    state Led_on
      en:
      warning_led=1;
    (default) -> Led_off
    Led_on -> Led_off : [after(1,sec)]
    Led_off -> Led_on : [after(1,sec)]
  (default) -> Cond_1
  Cond_1 -> Cond_2 : [Signal==0 && Current >1]
  Cond_2 -> Cond_1 : [Signal == 0 && Current <1 ]
  data: Current input; Signal input; relay_adhesive_fault output; warning_led output

== stateflow chart BMS_Advanced_Protection_Algorithm_Design/Advanced_Protection_Algorithm/Voltage_Protection/Cell_Under_Voltage_Protection/Under_Voltage_Protection ==
  state Initial_Condition
    en:
    Cell_Under_voltage_fault=0;
    Warning_led=0;
  state Level_1_Trigger
    en:
    Cell_Under_voltage_fault=1;
    state LED_off
      en:
      Warning_led=0;
    state LED_on
      en:
      Warning_led=1;
    (default) -> LED_off
    LED_off -> LED_on : [after(1,sec)]
    LED_on -> LED_off : [after(1,sec)]
  state Level_3_Trigger
    en:
    Cell_Under_voltage_fault=1;
    Warning_led=1;
    du:
    Warning_led=1;
  (default) -> Initial_Condition
  Initial_Condition -> Level_1_Trigger : [Cell_Voltage <3  && after(5,sec)]
  Level_1_Trigger -> Initial_Condition [order 1] : [Cell_Voltage > 3.05]
  Level_3_Trigger -> Initial_Condition [order 2] : [Cell_Voltage > 3.05]
  Level_1_Trigger -> Level_3_Trigger [order 2] : [Cell_Voltage < 2.8 && after(3,sec)]
  Level_3_Trigger -> Level_1_Trigger [order 1] : [Cell_Voltage > 2.85]
  data: Cell_Voltage input; Warning_led output; Cell_Under_voltage_fault output

== stateflow chart BMS_Advanced_Protection_Algorithm_Design/Advanced_Protection_Algorithm/Voltage_Protection/Pack_Over_Voltage_Protection/Over_Voltage_Protection ==
  state Initial_Condition
    en:
    Pack_over_voltage_fault=0;
    Warning_led=0;
  state Level_1_Trigger
    en:
    Pack_over_voltage_fault=1;
    state LED_off
      en:
      Warning_led=0;
    state LED_on
      en:
      Warning_led=1;
    (default) -> LED_off
    LED_off -> LED_on : [after(1,sec)]
    LED_on -> LED_off : [after(1,sec)]
  state Level_3_Trigger
    en:
    Pack_over_voltage_fault=1;
    Warning_led=1;
    du:
    Warning_led=1;
  (default) -> Initial_Condition
  Initial_Condition -> Level_1_Trigger : [Pack_Voltage > 56 && after(5,sec)]
  Level_1_Trigger -> Initial_Condition [order 1] : [Pack_Voltage < 55]
  Level_3_Trigger -> Initial_Condition [order 2] : [Pack_Voltage<55]
  Level_1_Trigger -> Level_3_Trigger [order 2] : [Pack_Voltage>58 && after(3,sec)]
  Level_3_Trigger -> Level_1_Trigger [order 1] : [Pack_Voltage<57.5]
  data: Warning_led output; Pack_Voltage input; Pack_over_voltage_fault output

== stateflow chart BMS_Advanced_Protection_Algorithm_Design/Advanced_Protection_Algorithm/Voltage_Protection/Cell_Over_Voltage_Protection/Over_Voltage_Protection ==
  state Initial_Condition
    en:
    Cell_over_voltage_fault=0;
    Warning_led=0;
  state Level_1_Trigger
    en:
    Cell_over_voltage_fault=1;
    state LED_off
      en:
      Warning_led=0;
    state LED_on
      en:
      Warning_led=1;
    (default) -> LED_off
    LED_off -> LED_on : [after(1,sec)]
    LED_on -> LED_off : [after(1,sec)]
  state Level_3_Trigger
    en:
    Cell_over_voltage_fault=1;
    Warning_led=1;
    du:
    Warning_led=1;
  (default) -> Initial_Condition
  Initial_Condition -> Level_1_Trigger : [Cell_Voltage > 4.15 && after(5,sec)]
  Level_1_Trigger -> Initial_Condition [order 1] : [Cell_Voltage < 4.13]
  Level_3_Trigger -> Initial_Condition [order 2] : [Cell_Voltage<4.13]
  Level_1_Trigger -> Level_3_Trigger [order 2] : [Cell_Voltage>4.22 && after(3,sec)]
  Level_3_Trigger -> Level_1_Trigger [order 1] : [Cell_Voltage<4.20]
  data: Cell_Voltage input; Warning_led output; Cell_over_voltage_fault output

== stateflow chart BMS_Advanced_Protection_Algorithm_Design/Advanced_Protection_Algorithm/Voltage_Protection/Pack_Under_Voltage_Protection/Under_Voltage_Protection ==
  state Initial_Condition
    en:
    Pack_Under_voltage_fault=0;
    Warning_led=0;
  state Level_1_Trigger
    en:
    Pack_Under_voltage_fault=1;
    state LED_off
      en:
      Warning_led=0;
    state LED_on
      en:
      Warning_led=1;
    (default) -> LED_off
    LED_off -> LED_on : [after(1,sec)]
    LED_on -> LED_off : [after(1,sec)]
  state Level_3_Trigger
    en:
    Pack_Under_voltage_fault=1;
    Warning_led=1;
    du:
    Warning_led=1;
  (default) -> Initial_Condition
  Initial_Condition -> Level_1_Trigger : [Pack_Voltage < 42 && after(5,sec)]
  Level_1_Trigger -> Initial_Condition [order 1] : [Pack_Voltage > 42.5]
  Level_3_Trigger -> Initial_Condition [order 2] : [Pack_Voltage > 42.5]
  Level_1_Trigger -> Level_3_Trigger [order 2] : [Pack_Voltage < 39.2 && after(3,sec)]
  Level_3_Trigger -> Level_1_Trigger [order 1] : [Pack_Voltage > 40]
  data: Warning_led output; Pack_Voltage input; Pack_Under_voltage_fault output
